simulink model "modelo_termico_completo"  (R2023b)
settings: Solver=VariableStepAuto  StartTime=0.0  StopTime=10.0  RelTol=1e-3
values from neighbouring files (symbols this model uses):
  alpha_cu = 3.9*10^-3    (= 0.0039)    [polos_y_ceros.m]    (also in var1.m)
  C_ts = 0.818    [polos_y_ceros.m]    (also in var1.m)
  R_sREF = 1.02    [polos_y_ceros.m]    (also in var1.m)
  R_ts_amb = 146.7    [polos_y_ceros.m]    (also in var1.m)
undefined symbols (not defined in the file or in its folder): magnitude
settings Model: Creator=tomas  LastModifiedBy=tomas

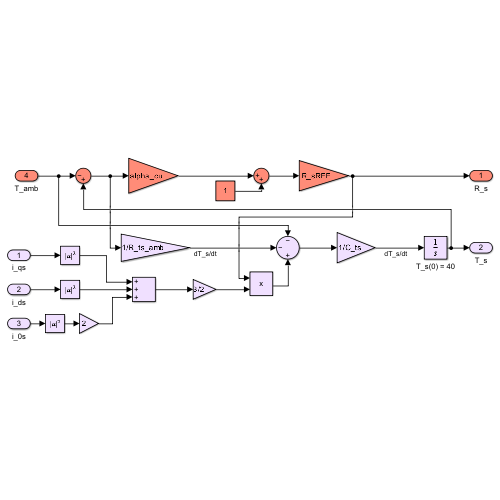
[thumbnail: Simulink's stored preview of the top-level diagram]
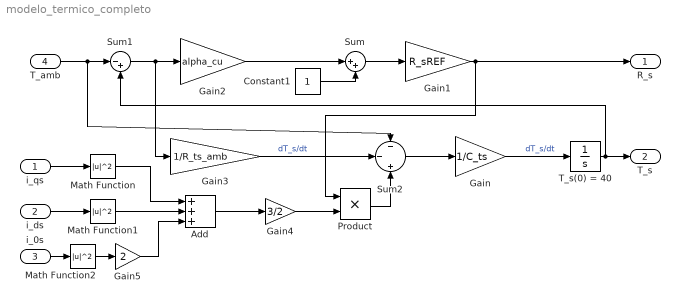
== system modelo_termico_completo ==
  i_qs : Inport
  i_ds : Inport  Port=2
  i_0s : Inport  Port=3
  T_amb : Inport  Port=4
  Add : Sum  Inputs=+++
  Constant1 : Constant
  Gain : Gain  Gain=1/C_ts
  Gain1 : Gain  Gain=R_sREF
  Gain2 : Gain  Gain=alpha_cu
  Gain3 : Gain  Gain=1/R_ts_amb
  Gain4 : Gain  Gain=3/2
  Gain5 : Gain  Gain=2
  Math Function : Math  Operator=magnitude^2
  Math Function1 : Math  Operator=magnitude^2
  Math Function2 : Math  Operator=magnitude^2
  Product : Product
  Sum : Sum  Inputs=|++
  Sum1 : Sum  Inputs=|-+
  Sum2 : Sum  Inputs=-|-|+
  T_s(0) = 40 : Integrator  InitialCondition=40
  R_s : Outport
  T_s : Outport  Port=2
  wires:
  Gain/1 -> T_s(0) = 40/1  "dT_s/dt"
  Gain1/1 -> Product/1, R_s/1
  Constant1/1 -> Sum/2
  T_s(0) = 40/1 -> T_s/1, Sum1/2
  T_amb/1 -> Sum2/1, Sum1/1
  Sum1/1 -> Gain3/1, Gain2/1
  Gain2/1 -> Sum/1
  Sum/1 -> Gain1/1
  Math Function/1 -> Add/1
  Math Function1/1 -> Add/2
  i_ds/1 -> Math Function1/1
  i_qs/1 -> Math Function/1
  Add/1 -> Gain4/1
  Gain4/1 -> Product/2
  i_0s/1 -> Math Function2/1
  Math Function2/1 -> Gain5/1
  Gain5/1 -> Add/3
  Product/1 -> Sum2/3
  Gain3/1 -> Sum2/2  "dT_s/dt"
  Sum2/1 -> Gain/1
